simulink model "test_bandpass"  (R2018b)
settings: Solver=ode4  StartTime=0.0  StopTime=0.12  FixedStep=0.01/44100  RelTol=1e-3
libraries: dsparch4 x1, commanapbnd3 x1
settings Model: Creator=HsuWeiChe  LastModifiedBy=HsuWeiChe

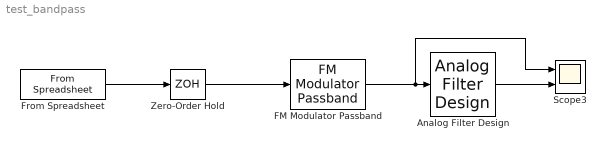
== system test_bandpass ==
  Analog Filter Design : dsparch4/Analog Filter Design  method=Butterworth  filttype=Bandpass  N=1  Wlo=2*pi*(1e06-1e05)  Whi=2*pi*(1e06+1e05)  Rp=2  Rs=40
  FM Modulator Passband : commanapbnd3/FM Modulator Passband  Fc=1e06  Ph=0  Kc=77017
      settings: SourceProductName=Communications System Toolbox  SourceProductBaseCode=CM
  From Spreadsheet : FromSpreadsheet  FileName=/Users/HsuWeiChe/Downloads/audiofile.xlsx  TreatFirstColumnAs=Data  SampleTime=1/44100
  Scope3 : Scope  NumInputPorts=2
  Zero-Order Hold : ZeroOrderHold  SampleTime=1/44100
  wires:
  FM Modulator Passband/1 -> Scope3/1, Analog Filter Design/1
  Analog Filter Design/1 -> Scope3/2
  From Spreadsheet/1 -> Zero-Order Hold/1
  Zero-Order Hold/1 -> FM Modulator Passband/1
